simulink model "simulation"  (R2019a)
settings: Solver=ode45  StartTime=0.0  StopTime=300  FixedStep=Ts  RelTol=1e-3  EnableMultiTasking=on
values from neighbouring files (symbols this model uses):
  Ad = M22'    [VanLoan.m]    (also in initKalmanFilter.m = N(11:20, 11:20)')
  alfa1 = .2    (= 0.2)    [parameters.m]
  alfa2 = .2    (= 0.2)    [parameters.m]
  b1 = 0.1    [createModelFile.m]    (also in initCtrlPlantModel.m; parameters.m)
  b2 = 0.1    [createModelFile.m]    (also in initCtrlPlantModel.m; parameters.m)
  b3_nom = 0.1    [parameters.m]
  b4_nom = 0.1    [parameters.m]
  b5 = 0.1    [createModelFile.m]    (also in initCtrlPlantModel.m; parameters.m)
  Bd = N12    [VanLoan.m]
  C_D_Re_GNARC = C_C_Re    [start_up.m]
  Cc = [ ... (first row only)    [initCtrlPlantModel.m]    (also in initKFs.m = ctrlPlantModel.C; initTask1.m = ctrlPlantModel.C)
  D_D_Re_GNARC = D_C_Re    [start_up.m]
  k1 = 0.15    [createModelFile.m]    (also in initCtrlPlantModel.m; parameters.m)
  k3_nom = .1    (= 0.1)    [parameters.m]
  k4_nom = .1    (= 0.1)    [parameters.m]
  m1 = 1    [parameters.m]
  m2 = 1    [parameters.m]
  m3 = 1    [parameters.m]
  m4 = 1    [parameters.m]
  P0 = diag([1, 1, 1, 1, 10, 10, 10, 10, 1, 1].^2)    [initKFs.m]    (also in initTask1.m = diag([1e-3, 1e-3, 1e-3, 1e-3, 1e-3, 1e-3, 1e-3, 1e-3, 1e-3, ; initTask2.m = diag([1e-3, 1e-3, 1e-3, 1e-3, 1e-3, 1e-3, 1e-3, 1e-3, 1e-3, )
  probThreshold = 1e-6    (= 1e-06)    [initTask2.m]
  Qd = M22'*M12    [VanLoan.m]    (also in initKalmanFilter.m = Ad*N(1:10, 11:20))
  Rd = R / Ts    [initKFs.m]    (also in initTask1.m = Rn / Ts; initTask2.m = Rn / Ts)
  Ts = .001    (= 0.001)    [parameters.m]
  x0 = [0; 0; 0; 0; 0; 0; 0; 0; 0; 0;]    [initKFs.m]    (also in initTask1.m; initTask2.m)
undefined symbols (not defined in the file or in its folder): A_D_Re_GNARC, Ad1, Ad2, Ad3, B_D_Re_GNARC, Bd1, Bd2, Bd3, L1, L2, L3, P1, P2, P3, Qd1, Qd2, Qd3
libraries: simulink x4
settings Model: Creator=VAHiD  LastModifiedBy=marti
settings DataIOCC: LimitDataPoints=on  SaveFormat=Array  ReturnWorkspaceOutputs=off
settings OptimizationCC: ExpressionDepthLimit=2147483647  LifeSpan=inf
settings DebuggingCC: UnderspecifiedInitializationDetection=Classic  MergeDetectMultiDrivingBlocksExec=none  SolverPrmCheckMsg=warning  FcnCallInpInsideContextMsg=warning  StateNameClashWarn=warning  PregeneratedLibrarySubsystemCodeDiagnostic=none  SFUnexpectedBacktrackingDiag=warning  SFNoUnconditionalDefaultTransitionDiag=warning  SFExecutionAtInitializationDiag=none  ArithmeticOperatorsInVariantConditions=warning
settings HardwareCC: ProdBitPerPointer=32  ProdBitPerSizeT=32  ProdBitPerPtrDiffT=32  ProdLargestAtomicFloat=None  ProdIntDivRoundTo=Undefined  ProdEndianess=Unspecified  ProdWordSize=32  ProdHWDeviceType=32-bit Generic
settings ModelReferenceCC: PropagateSignalLabelsOutOfModel=off
settings SFSimCC: SimUseLocalCustomCode=off
settings RTWCC: RTWUseLocalCustomCode=off
settings CodeAppCC: StateflowObjectComments=on
settings GRTTargetCC: TargetLangStandard=C89/C90 (ANSI)  GeneratePreprocessorConditionals=Disable all  CombineOutputUpdateFcns=off  GRTInterface=on
settings ConfigComp: CovMetricSettings=dw  CovHtmlReporting=on  CovSaveCumulativeToWorkspaceVar=on  CovSaveSingleToWorkspaceVar=on  CovExternalEMLEnable=off

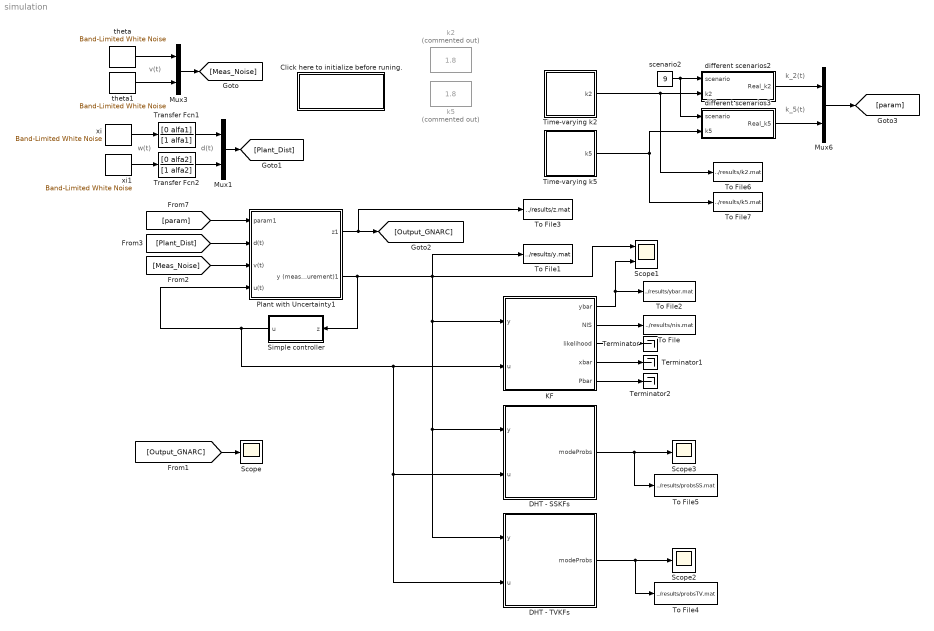
== system simulation ==
  note: w(t)
  note: v(t)
  note: d(t)
  note: k_2(t)
  note: k_5(t)
  Click here to initialize before runing. : Subsystem
      settings: OpenFcn=start_up
      mask Display: disp('Load\Parameters')
  DHT - SSKFs : Subsystem
  DHT - TVKFs : Subsystem
  KF : Subsystem
  Mux1 : Mux  Inputs=2
  Mux3 : Mux  Inputs=2
  Mux6 : Mux  Inputs=2
  Plant with Uncertainty1 : Subsystem
  Scope : Scope
  Scope1 : Scope  NumInputPorts=2
  Scope2 : Scope
  Scope3 : Scope
  Simple controller : Subsystem
  Terminator : Terminator
  Terminator1 : Terminator
  Terminator2 : Terminator
  Time-varying k2 : Subsystem
  Time-varying k5 : Subsystem
  To File : ToFile  Filename=../results/nis.mat  MatrixName=nis
  To File1 : ToFile  Filename=../results/y.mat  MatrixName=y
  To File2 : ToFile  Filename=../results/ybar.mat  MatrixName=ybar
  To File3 : ToFile  Filename=../results/z.mat  MatrixName=z
  To File4 : ToFile  Filename=../results/probsTV.mat  MatrixName=probsTV
  To File5 : ToFile  Filename=../results/probsSS.mat  MatrixName=probsSS
  To File6 : ToFile  Filename=../results/k2.mat  MatrixName=k2
  To File7 : ToFile  Filename=../results/k5.mat  MatrixName=k5
  Transfer Fcn1 : TransferFcn  Numerator=[0 alfa1]  Denominator=[1 alfa1]
  Transfer Fcn2 : TransferFcn  Numerator=[0 alfa2]  Denominator=[1 alfa2]
  different scenarios2 : Subsystem
  different scenarios3 : Subsystem
  k2 : Constant  Commented=on  Value=1.8
  k5 : Constant  Commented=on  Value=1.8
  scenario2 : Constant  Value=9
  theta : simulink/Sources/Band-Limited White Noise  Cov=TH1  Ts=Ts  seed=1
  theta1 : simulink/Sources/Band-Limited White Noise  Cov=TH2  Ts=Ts  seed=2
  xi : simulink/Sources/Band-Limited White Noise  Cov=XI1  Ts=Ts  seed=3
  xi1 : simulink/Sources/Band-Limited White Noise  Cov=XI2  Ts=Ts  seed=4
  wires:
  Mux3/1 -> [Meas_Noise]
  theta/1 -> Mux3/1
  theta1/1 -> Mux3/2
  Mux1/1 -> [Plant_Dist]
  xi/1 -> Transfer Fcn1/1
  xi1/1 -> Transfer Fcn2/1
  Transfer Fcn1/1 -> Mux1/1
  Transfer Fcn2/1 -> Mux1/2
  scenario2/1 -> different scenarios2/1(scenario), different scenarios3/1(scenario)
  different scenarios3/1(Real_k5) -> Mux6/2
  different scenarios2/1(Real_k2) -> Mux6/1
  Mux6/1 -> [param]
  [param] -> Plant with Uncertainty1/1(param1)
  [Plant_Dist] -> Plant with Uncertainty1/2(d(t))
  [Meas_Noise] -> Plant with Uncertainty1/3(v(t))
  Plant with Uncertainty1/1(z1) -> To File3/1, [Output_GNARC]
  Simple controller/1(u) -> DHT - SSKFs/2(u), DHT - TVKFs/2(u), KF/2(u), Plant with Uncertainty1/4(u(t))
  [Output_GNARC] -> Scope/1
  Plant with Uncertainty1/2(y (measurement)1) -> Simple controller/1(z), DHT - TVKFs/1(y), DHT - SSKFs/1(y), KF/1(y), Scope1/1, To File1/1
  KF/4(xbar) -> Terminator1/1
  KF/3(likelihood) -> Terminator/1
  KF/5(Pbar) -> Terminator2/1
  KF/1(ybar) -> To File2/1, Scope1/2
  KF/2(NIS) -> To File/1
  DHT - TVKFs/1(modeProbs) -> Scope2/1, To File4/1
  DHT - SSKFs/1(modeProbs) -> To File5/1, Scope3/1
  Time-varying k2/1(k2) -> To File6/1, different scenarios2/2(k2)
  Time-varying k5/1(k5) -> To File7/1, different scenarios3/2(k5)

== system simulation/Click here to initialize before runing. ==

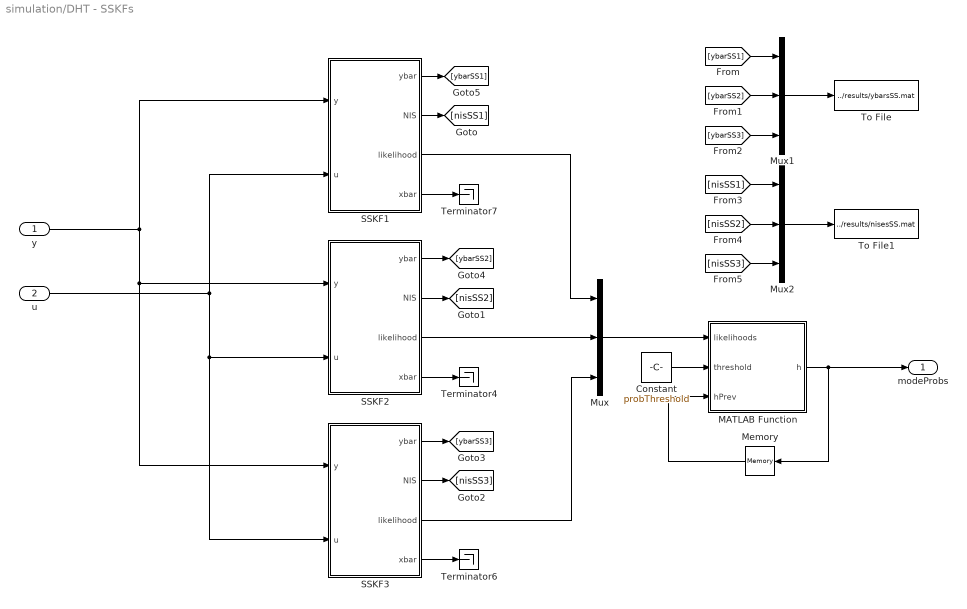
== system simulation/DHT - SSKFs ==
  y : Inport
  u : Inport  Port=2
  Constant : Constant  Value=probThreshold
  MATLAB Function : MATLAB Function  TreatAsAtomicUnit=on
  Memory : Memory  InitialCondition=[1/3, 1/3, 1/3]
  Mux : Mux  Inputs=3
  Mux1 : Mux  Inputs=3
  Mux2 : Mux  Inputs=3
  SSKF1 : Subsystem
  SSKF2 : Subsystem
  SSKF3 : Subsystem
  Terminator4 : Terminator
  Terminator6 : Terminator
  Terminator7 : Terminator
  To File : ToFile  Filename=../results/ybarsSS.mat  MatrixName=ybarsSS
  To File1 : ToFile  Filename=../results/nisesSS.mat  MatrixName=nisesSS
  modeProbs : Outport
  wires:
  u/1 -> SSKF3/2(u), SSKF2/2(u), SSKF1/2(u)
  y/1 -> SSKF3/1(y), SSKF2/1(y), SSKF1/1(y)
  SSKF1/3(likelihood) -> Mux/1
  SSKF2/3(likelihood) -> Mux/2
  SSKF3/3(likelihood) -> Mux/3
  SSKF2/1(ybar) -> [ybarSS2]
  SSKF1/1(ybar) -> [ybarSS1]
  SSKF1/2(NIS) -> [nisSS1]
  SSKF2/2(NIS) -> [nisSS2]
  SSKF3/1(ybar) -> [ybarSS3]
  SSKF2/4(xbar) -> Terminator4/1
  SSKF3/4(xbar) -> Terminator6/1
  SSKF1/4(xbar) -> Terminator7/1
  SSKF3/2(NIS) -> [nisSS3]
  Constant/1 -> MATLAB Function/2(threshold)
  MATLAB Function/1(h) -> modeProbs/1, Memory/1
  Memory/1 -> MATLAB Function/3(hPrev)
  Mux/1 -> MATLAB Function/1(likelihoods)
  [ybarSS1] -> Mux1/1
  [ybarSS2] -> Mux1/2
  [ybarSS3] -> Mux1/3
  Mux1/1 -> To File/1
  [nisSS2] -> Mux2/2
  [nisSS3] -> Mux2/3
  [nisSS1] -> Mux2/1
  Mux2/1 -> To File1/1

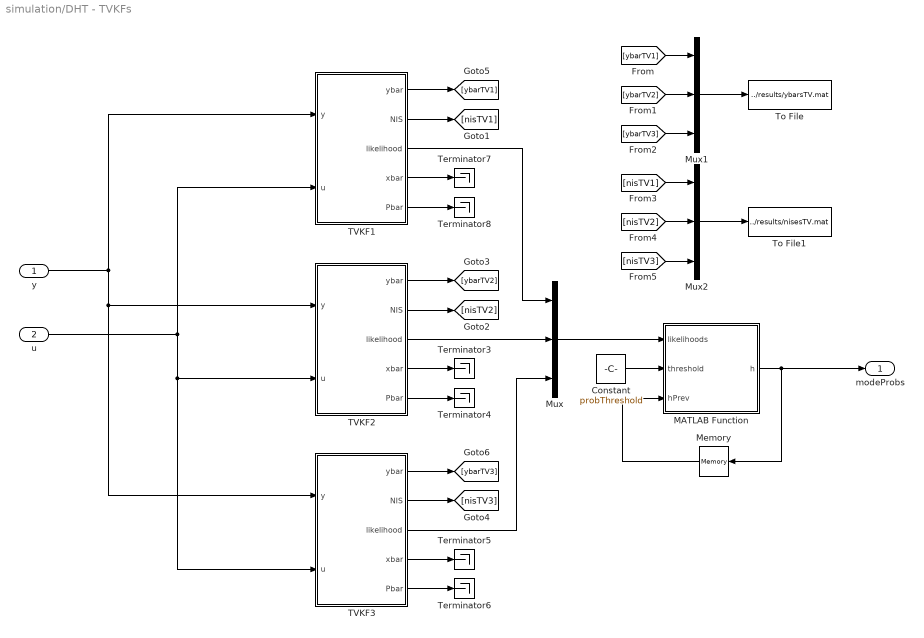
== system simulation/DHT - TVKFs ==
  y : Inport
  u : Inport  Port=2
  Constant : Constant  Value=probThreshold
  MATLAB Function : MATLAB Function  TreatAsAtomicUnit=on
  Memory : Memory  InitialCondition=[1/3, 1/3, 1/3]
  Mux : Mux  Inputs=3
  Mux1 : Mux  Inputs=3
  Mux2 : Mux  Inputs=3
  TVKF1 : Subsystem
  TVKF2 : Subsystem
  TVKF3 : Subsystem
  Terminator{3..8} (6 alike) : Terminator
  To File : ToFile  Filename=../results/ybarsTV.mat  MatrixName=ybarsTV
  To File1 : ToFile  Filename=../results/nisesTV.mat  MatrixName=nisesTV
  modeProbs : Outport
  wires:
  u/1 -> TVKF3/2(u), TVKF2/2(u), TVKF1/2(u)
  y/1 -> TVKF3/1(y), TVKF2/1(y), TVKF1/1(y)
  TVKF1/3(likelihood) -> Mux/1
  TVKF2/3(likelihood) -> Mux/2
  TVKF3/3(likelihood) -> Mux/3
  Mux/1 -> MATLAB Function/1(likelihoods)
  MATLAB Function/1(h) -> modeProbs/1, Memory/1
  Memory/1 -> MATLAB Function/3(hPrev)
  TVKF3/1(ybar) -> [ybarTV3]
  TVKF2/1(ybar) -> [ybarTV2]
  TVKF1/1(ybar) -> [ybarTV1]
  TVKF1/2(NIS) -> [nisTV1]
  TVKF2/2(NIS) -> [nisTV2]
  TVKF3/2(NIS) -> [nisTV3]
  TVKF2/4(xbar) -> Terminator3/1
  TVKF2/5(Pbar) -> Terminator4/1
  TVKF3/4(xbar) -> Terminator5/1
  TVKF3/5(Pbar) -> Terminator6/1
  TVKF1/4(xbar) -> Terminator7/1
  TVKF1/5(Pbar) -> Terminator8/1
  Constant/1 -> MATLAB Function/2(threshold)
  Mux1/1 -> To File/1
  [nisTV1] -> Mux2/1
  [ybarTV3] -> Mux1/3
  [ybarTV1] -> Mux1/1
  [nisTV3] -> Mux2/3
  Mux2/1 -> To File1/1
  [ybarTV2] -> Mux1/2
  [nisTV2] -> Mux2/2

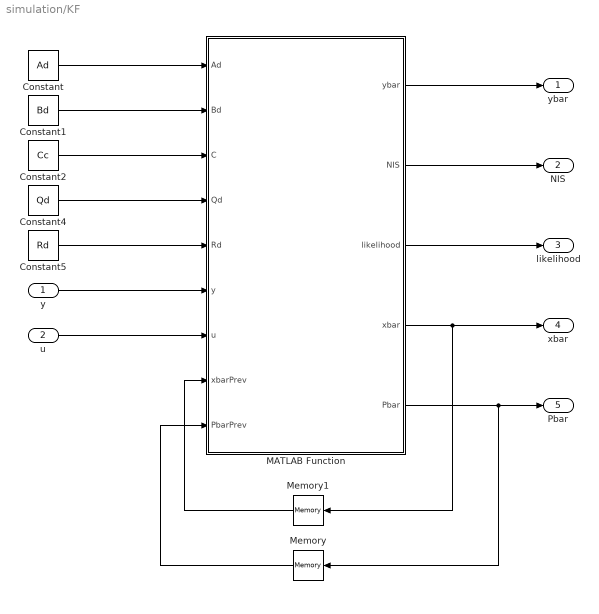
== system simulation/KF ==
  y : Inport
  u : Inport  Port=2
  Constant : Constant  Value=Ad
  Constant1 : Constant  Value=Bd
  Constant2 : Constant  Value=Cc
  Constant4 : Constant  Value=Qd
  Constant5 : Constant  Value=Rd
  MATLAB Function : MATLAB Function  TreatAsAtomicUnit=on
  Memory : Memory  InitialCondition=P0
  Memory1 : Memory  InitialCondition=x0
  ybar : Outport
  NIS : Outport  Port=2
  likelihood : Outport  Port=3
  xbar : Outport  Port=4
  Pbar : Outport  Port=5
  wires:
  y/1 -> MATLAB Function/6(y)
  u/1 -> MATLAB Function/7(u)
  MATLAB Function/1(ybar) -> ybar/1
  Constant2/1 -> MATLAB Function/3(C)
  Constant1/1 -> MATLAB Function/2(Bd)
  Constant/1 -> MATLAB Function/1(Ad)
  Constant4/1 -> MATLAB Function/4(Qd)
  Constant5/1 -> MATLAB Function/5(Rd)
  MATLAB Function/2(NIS) -> NIS/1
  MATLAB Function/3(likelihood) -> likelihood/1
  MATLAB Function/4(xbar) -> Memory1/1, xbar/1
  MATLAB Function/5(Pbar) -> Memory/1, Pbar/1
  Memory1/1 -> MATLAB Function/8(xbarPrev)
  Memory/1 -> MATLAB Function/9(PbarPrev)

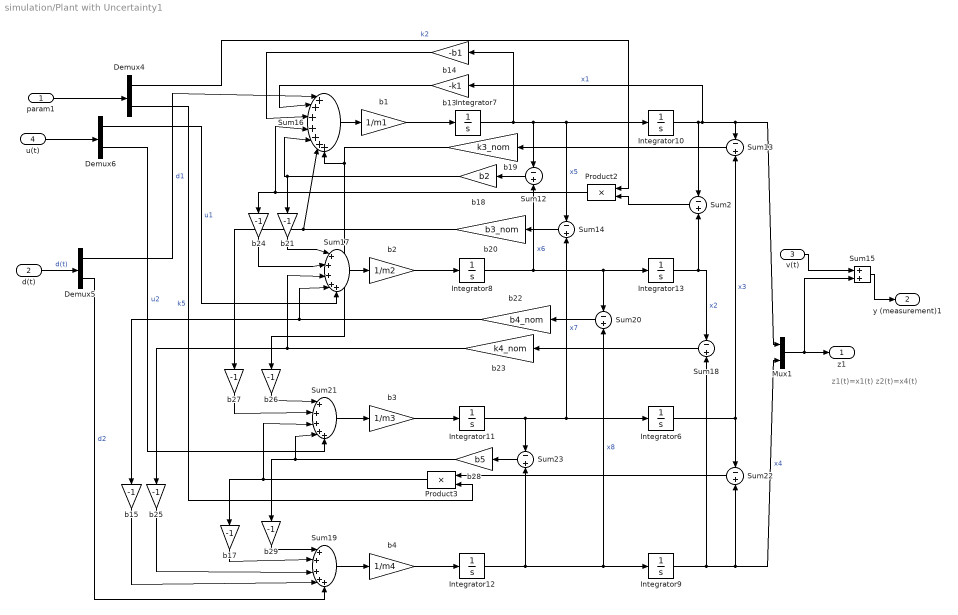
== system simulation/Plant with Uncertainty1 ==
  note: z1(t)=x1(t)
      | z2(t)=x4(t)
  param1 : Inport
  d(t) : Inport  Port=2
  v(t) : Inport  Port=3
  u(t) : Inport  Port=4
  Demux4 : Demux  Outputs=2
  Demux5 : Demux  Outputs=2
  Demux6 : Demux  Outputs=2
  Integrator{6..13} (8 alike) : Integrator
  Mux1 : Mux  Inputs=2
  Product2 : Product  SaturateOnIntegerOverflow=on  InputSameDT=on  OutDataTypeStr=Inherit: Same as first input
  Product3 : Product  SaturateOnIntegerOverflow=on  InputSameDT=on  OutDataTypeStr=Inherit: Same as first input
  Sum{2,12..14,18,20,22..23} (8 alike) : Sum  Inputs=-+  SaturateOnIntegerOverflow=on  InputSameDT=on  OutDataTypeStr=Inherit: Same as first input
  Sum15 : Sum  SaturateOnIntegerOverflow=on  InputSameDT=on  OutDataTypeStr=Inherit: Same as first input
  Sum16 : Sum  Inputs=|+++++++  SaturateOnIntegerOverflow=on  InputSameDT=on  OutDataTypeStr=Inherit: Same as first input
  Sum17 : Sum  Inputs=|+++++  SaturateOnIntegerOverflow=on  InputSameDT=on  OutDataTypeStr=Inherit: Same as first input
  Sum19 : Sum  Inputs=|+++++  SaturateOnIntegerOverflow=on  InputSameDT=on  OutDataTypeStr=Inherit: Same as first input
  Sum21 : Sum  Inputs=|+++++  SaturateOnIntegerOverflow=on  InputSameDT=on  OutDataTypeStr=Inherit: Same as first input
  b1 : Gain  Gain=1/m1  SaturateOnIntegerOverflow=on  OutDataTypeStr=Inherit: Same as input  ParamDataTypeStr=Inherit: Same as input
  b13 : Gain  Gain=-k1  SaturateOnIntegerOverflow=on  OutDataTypeStr=Inherit: Same as input  ParamDataTypeStr=Inherit: Same as input
  b14 : Gain  Gain=-b1  SaturateOnIntegerOverflow=on  OutDataTypeStr=Inherit: Same as input  ParamDataTypeStr=Inherit: Same as input
  b{15,17,21,24..27,29} (8 alike) : Gain  Gain=-1  SaturateOnIntegerOverflow=on  OutDataTypeStr=Inherit: Same as input  ParamDataTypeStr=Inherit: Same as input
  b18 : Gain  Gain=b2  SaturateOnIntegerOverflow=on  OutDataTypeStr=Inherit: Same as input  ParamDataTypeStr=Inherit: Same as input
  b19 : Gain  Gain=k3_nom  SaturateOnIntegerOverflow=on  OutDataTypeStr=Inherit: Same as input  ParamDataTypeStr=Inherit: Same as input
  b2 : Gain  Gain=1/m2  SaturateOnIntegerOverflow=on  OutDataTypeStr=Inherit: Same as input  ParamDataTypeStr=Inherit: Same as input
  b20 : Gain  Gain=b3_nom  SaturateOnIntegerOverflow=on  OutDataTypeStr=Inherit: Same as input  ParamDataTypeStr=Inherit: Same as input
  b22 : Gain  Gain=b4_nom  SaturateOnIntegerOverflow=on  OutDataTypeStr=Inherit: Same as input  ParamDataTypeStr=Inherit: Same as input
  b23 : Gain  Gain=k4_nom  SaturateOnIntegerOverflow=on  OutDataTypeStr=Inherit: Same as input  ParamDataTypeStr=Inherit: Same as input
  b28 : Gain  Gain=b5  SaturateOnIntegerOverflow=on  OutDataTypeStr=Inherit: Same as input  ParamDataTypeStr=Inherit: Same as input
  b3 : Gain  Gain=1/m3  SaturateOnIntegerOverflow=on  OutDataTypeStr=Inherit: Same as input  ParamDataTypeStr=Inherit: Same as input
  b4 : Gain  Gain=1/m4  SaturateOnIntegerOverflow=on  OutDataTypeStr=Inherit: Same as input  ParamDataTypeStr=Inherit: Same as input
  z1 : Outport
  y (measurement)1 : Outport  Port=2
  wires:
  Sum15/1 -> y (measurement)1/1
  v(t)/1 -> Sum15/1
  param1/1 -> Demux4/1
  Mux1/1 -> Sum15/2, z1/1
  d(t)/1 -> Demux5/1  "d(t)"
  u(t)/1 -> Demux6/1
  b25/1 -> Sum19/3
  b15/1 -> Sum19/4
  Demux5/2 -> Sum19/5  "d2"
  Integrator7/1 -> b14/1, Sum12/1, Integrator10/1, Sum14/1  "x5"
  Integrator10/1 -> b13/1, Sum13/1, Mux1/1, Sum2/1  "x1"
  Integrator8/1 -> Sum12/2, Integrator13/1, Sum20/1  "x6"
  Integrator11/1 -> Integrator6/1, Sum14/2, Sum23/1  "x7"
  Integrator12/1 -> Integrator9/1, Sum20/2, Sum23/2  "x8"
  Demux5/1 -> Sum16/1  "d1"
  b13/1 -> Sum16/2
  b14/1 -> Sum16/3
  Integrator13/1 -> Sum2/2, Sum18/1  "x2"
  Sum2/1 -> Product2/2
  Demux4/1 -> Product2/1  "k2"
  Sum12/1 -> b18/1
  b18/1 -> Sum16/5, b21/1
  Integrator6/1 -> Sum13/2, Sum22/1  "x3"
  Sum13/1 -> b19/1
  Sum14/1 -> b20/1
  b20/1 -> Sum16/6, b27/1
  Sum16/1 -> b1/1
  Product2/1 -> Sum16/4, b24/1
  Integrator9/1 -> Sum18/2, Sum22/2, Mux1/2  "x4"
  Sum18/1 -> b23/1
  b23/1 -> Sum17/3, b25/1
  Sum17/1 -> b2/1
  Sum20/1 -> b22/1
  b22/1 -> Sum17/4, b15/1
  b21/1 -> Sum17/1
  b24/1 -> Sum17/2
  Demux6/1 -> Sum17/5  "u1"
  Sum21/1 -> b3/1
  b19/1 -> Sum16/7, b26/1
  b26/1 -> Sum21/1
  b27/1 -> Sum21/2
  Sum22/1 -> Product3/1
  Product3/1 -> Sum21/3, b17/1
  Demux4/2 -> Product3/2  "k5"
  Sum23/1 -> b28/1
  b28/1 -> Sum21/4, b29/1
  Demux6/2 -> Sum21/5  "u2"
  Sum19/1 -> b4/1
  b17/1 -> Sum19/2
  b29/1 -> Sum19/1
  b1/1 -> Integrator7/1
  b2/1 -> Integrator8/1
  b3/1 -> Integrator11/1
  b4/1 -> Integrator12/1

== system simulation/Simple controller ==
  z : Inport
  Discrete mu-controller 1 : DiscreteStateSpace  Description=disp('sss')  A=A_D_Re_GNARC  B=B_D_Re_GNARC  C=C_D_Re_GNARC  D=D_D_Re_GNARC  SampleTime=Ts
  u : Outport
  wires:
  z/1 -> Discrete mu-controller 1/1
  Discrete mu-controller 1/1 -> u/1

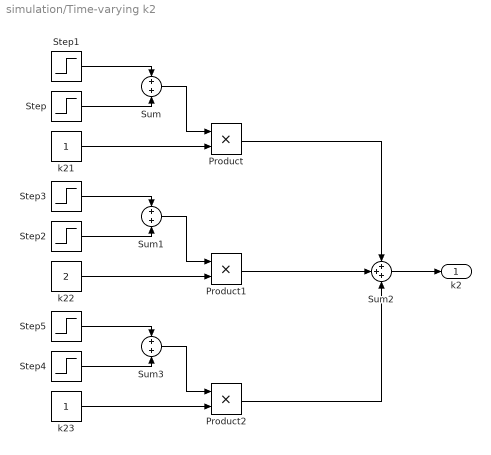
== system simulation/Time-varying k2 ==
  Product : Product
  Product1 : Product
  Product2 : Product
  Step : Step  Time=100  After=-1  SampleTime=0
  Step1 : Step  SampleTime=0
  Step2 : Step  Time=300  After=-1  SampleTime=0
  Step3 : Step  Time=100  SampleTime=0
  Step4 : Step  Time=300  After=-1  SampleTime=0
  Step5 : Step  Time=300  SampleTime=0
  Sum : Sum  Inputs=+|+
  Sum1 : Sum  Inputs=+|+
  Sum2 : Sum  Inputs=+++
  Sum3 : Sum  Inputs=+|+
  k21 : Constant
  k22 : Constant  Value=2
  k23 : Constant
  k2 : Outport
  wires:
  k21/1 -> Product/2
  Sum/1 -> Product/1
  Step1/1 -> Sum/1
  Step/1 -> Sum/2
  Step3/1 -> Sum1/1
  Sum1/1 -> Product1/1
  Step2/1 -> Sum1/2
  k22/1 -> Product1/2
  Sum3/1 -> Product2/1
  Step4/1 -> Sum3/2
  k23/1 -> Product2/2
  Step5/1 -> Sum3/1
  Product1/1 -> Sum2/2
  Product2/1 -> Sum2/3
  Product/1 -> Sum2/1
  Sum2/1 -> k2/1

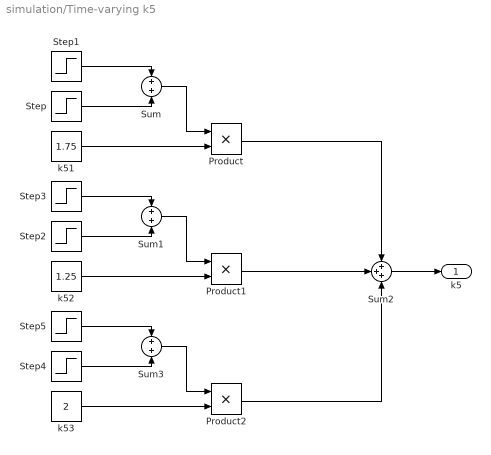
== system simulation/Time-varying k5 ==
  Product : Product
  Product1 : Product
  Product2 : Product
  Step : Step  Time=100  After=-1  SampleTime=0
  Step1 : Step  SampleTime=0
  Step2 : Step  Time=200  After=-1  SampleTime=0
  Step3 : Step  Time=100  SampleTime=0
  Step4 : Step  Time=300  After=-1  SampleTime=0
  Step5 : Step  Time=200  SampleTime=0
  Sum : Sum  Inputs=+|+
  Sum1 : Sum  Inputs=+|+
  Sum2 : Sum  Inputs=+++
  Sum3 : Sum  Inputs=+|+
  k51 : Constant  Value=1.75
  k52 : Constant  Value=1.25
  k53 : Constant  Value=2
  k5 : Outport
  wires:
  k51/1 -> Product/2
  Sum/1 -> Product/1
  Step1/1 -> Sum/1
  Step/1 -> Sum/2
  Step3/1 -> Sum1/1
  Sum1/1 -> Product1/1
  Step2/1 -> Sum1/2
  k52/1 -> Product1/2
  Sum3/1 -> Product2/1
  Step4/1 -> Sum3/2
  k53/1 -> Product2/2
  Step5/1 -> Sum3/1
  Product1/1 -> Sum2/2
  Product2/1 -> Sum2/3
  Product/1 -> Sum2/1
  Sum2/1 -> k5/1

== system simulation/different scenarios2 ==
  scenario : Inport
  k2 : Inport  Port=2
  GNARC : Sin  Amplitude=.75  Bias=1  Frequency=2*pi/700  Phase=-pi/2  SampleTime=0
  LNARC1 : Sin  Amplitude=.875  Bias=1.625  Frequency=2*pi/700  Phase=-pi/2  SampleTime=0
  LNARC2 : Sin  Amplitude=.55/2  Bias=.775  Frequency=2*pi/700  Phase=-pi/2  SampleTime=0
  LNARC3 : Sin  Amplitude=.75/2  Bias=1.4250  Frequency=2*pi/700  Phase=-pi/2  SampleTime=0
  LNARC4 : Sin  Amplitude=.15/2  Bias=.325  Frequency=2*pi/700  Phase=-pi/2  SampleTime=0
  LNARC5 : Sin  Amplitude=.15  Bias=.55  Frequency=2*pi/700  Phase=-pi/2  SampleTime=0
  LNARC6 : Sin  Amplitude=.45/2  Bias=.925  Frequency=2*pi/700  Phase=-pi/2  SampleTime=0
  LNARC7 : Sin  Amplitude=.30  Bias=1.45  Frequency=2*pi/700  Phase=-pi/2  SampleTime=0
  Multiport Switch : MultiPortSwitch  Inputs=9
  Real_k2 : Outport
  wires:
  Multiport Switch/1 -> Real_k2/1
  scenario/1 -> Multiport Switch/1
  LNARC3/1 -> Multiport Switch/4
  LNARC6/1 -> Multiport Switch/7
  LNARC7/1 -> Multiport Switch/8
  LNARC5/1 -> Multiport Switch/6
  LNARC4/1 -> Multiport Switch/5
  LNARC1/1 -> Multiport Switch/2
  LNARC2/1 -> Multiport Switch/3
  k2/1 -> Multiport Switch/10
  GNARC/1 -> Multiport Switch/9

== system simulation/different scenarios3 ==
  scenario : Inport
  k5 : Inport  Port=2
  GNARC : Sin  Amplitude=1.6  Bias=1.8  Frequency=2*pi/700  Phase=-pi/2  SampleTime=0
  LNARC1 : Sin  Amplitude=.8  Bias=1.7  Frequency=2*pi/700  Phase=-3*pi/2  SampleTime=0
  LNARC2 : Sin  Amplitude=.8  Bias=2.6  Frequency=2*pi/700  Phase=-pi/2  SampleTime=0
  LNARC3 : Sin  Amplitude=.8  Bias=2.6  Frequency=2*pi/700  Phase=-pi/2  SampleTime=0
  LNARC{4..7} (4 alike) : Sin  Amplitude=.8  Bias=1  Frequency=2*pi/700  Phase=-pi/2  SampleTime=0
  Multiport Switch : MultiPortSwitch  Inputs=9
  Real_k5 : Outport
  wires:
  LNARC5/1 -> Multiport Switch/6
  LNARC7/1 -> Multiport Switch/8
  LNARC6/1 -> Multiport Switch/7
  LNARC3/1 -> Multiport Switch/4
  scenario/1 -> Multiport Switch/1
  Multiport Switch/1 -> Real_k5/1
  k5/1 -> Multiport Switch/10
  GNARC/1 -> Multiport Switch/9
  LNARC1/1 -> Multiport Switch/2
  LNARC2/1 -> Multiport Switch/3
  LNARC4/1 -> Multiport Switch/5

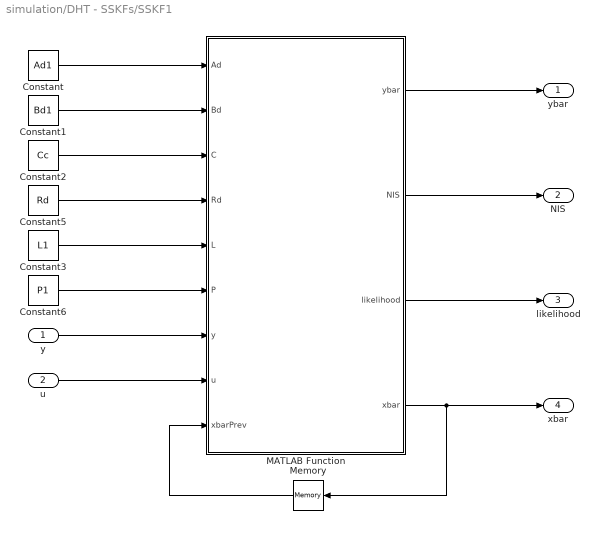
== system simulation/DHT - SSKFs/SSKF1 ==
  y : Inport
  u : Inport  Port=2
  Constant : Constant  Value=Ad1
  Constant1 : Constant  Value=Bd1
  Constant2 : Constant  Value=Cc
  Constant3 : Constant  Value=L1
  Constant5 : Constant  Value=Rd
  Constant6 : Constant  Value=P1
  MATLAB Function : MATLAB Function  TreatAsAtomicUnit=on
  Memory : Memory  InitialCondition=x0
  ybar : Outport
  NIS : Outport  Port=2
  likelihood : Outport  Port=3
  xbar : Outport  Port=4
  wires:
  y/1 -> MATLAB Function/7(y)
  u/1 -> MATLAB Function/8(u)
  MATLAB Function/1(ybar) -> ybar/1
  Constant2/1 -> MATLAB Function/3(C)
  Constant1/1 -> MATLAB Function/2(Bd)
  Constant/1 -> MATLAB Function/1(Ad)
  Constant5/1 -> MATLAB Function/4(Rd)
  MATLAB Function/2(NIS) -> NIS/1
  MATLAB Function/3(likelihood) -> likelihood/1
  MATLAB Function/4(xbar) -> xbar/1, Memory/1
  Constant3/1 -> MATLAB Function/5(L)
  Constant6/1 -> MATLAB Function/6(P)
  Memory/1 -> MATLAB Function/9(xbarPrev)

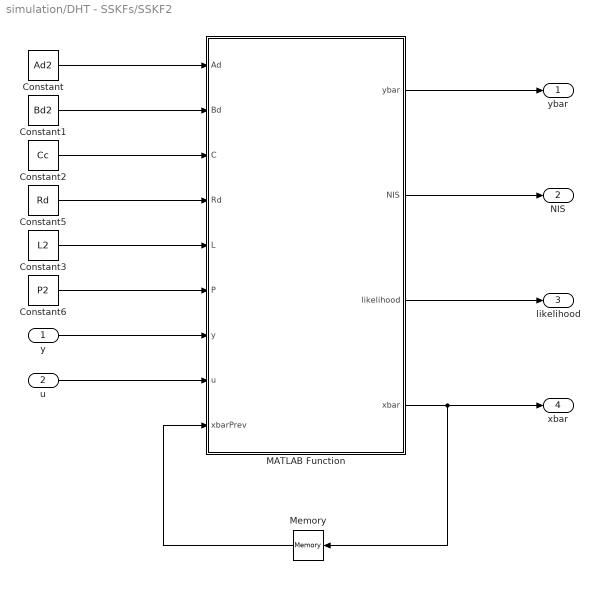
== system simulation/DHT - SSKFs/SSKF2 ==
  y : Inport
  u : Inport  Port=2
  Constant : Constant  Value=Ad2
  Constant1 : Constant  Value=Bd2
  Constant2 : Constant  Value=Cc
  Constant3 : Constant  Value=L2
  Constant5 : Constant  Value=Rd
  Constant6 : Constant  Value=P2
  MATLAB Function : MATLAB Function  TreatAsAtomicUnit=on
  Memory : Memory  InitialCondition=x0
  ybar : Outport
  NIS : Outport  Port=2
  likelihood : Outport  Port=3
  xbar : Outport  Port=4
  wires:
  y/1 -> MATLAB Function/7(y)
  u/1 -> MATLAB Function/8(u)
  MATLAB Function/1(ybar) -> ybar/1
  Constant2/1 -> MATLAB Function/3(C)
  Constant1/1 -> MATLAB Function/2(Bd)
  Constant/1 -> MATLAB Function/1(Ad)
  Constant5/1 -> MATLAB Function/4(Rd)
  MATLAB Function/2(NIS) -> NIS/1
  MATLAB Function/3(likelihood) -> likelihood/1
  MATLAB Function/4(xbar) -> xbar/1, Memory/1
  Constant3/1 -> MATLAB Function/5(L)
  Constant6/1 -> MATLAB Function/6(P)
  Memory/1 -> MATLAB Function/9(xbarPrev)

== system simulation/DHT - SSKFs/SSKF3 ==
  y : Inport
  u : Inport  Port=2
  Constant : Constant  Value=Ad3
  Constant1 : Constant  Value=Bd3
  Constant2 : Constant  Value=Cc
  Constant3 : Constant  Value=L3
  Constant5 : Constant  Value=Rd
  Constant6 : Constant  Value=P3
  MATLAB Function : MATLAB Function  TreatAsAtomicUnit=on
  Memory : Memory  InitialCondition=x0
  ybar : Outport
  NIS : Outport  Port=2
  likelihood : Outport  Port=3
  xbar : Outport  Port=4
  wires:
  y/1 -> MATLAB Function/7(y)
  u/1 -> MATLAB Function/8(u)
  MATLAB Function/1(ybar) -> ybar/1
  Constant2/1 -> MATLAB Function/3(C)
  Constant1/1 -> MATLAB Function/2(Bd)
  Constant/1 -> MATLAB Function/1(Ad)
  Constant5/1 -> MATLAB Function/4(Rd)
  MATLAB Function/2(NIS) -> NIS/1
  MATLAB Function/3(likelihood) -> likelihood/1
  MATLAB Function/4(xbar) -> xbar/1, Memory/1
  Constant3/1 -> MATLAB Function/5(L)
  Constant6/1 -> MATLAB Function/6(P)
  Memory/1 -> MATLAB Function/9(xbarPrev)

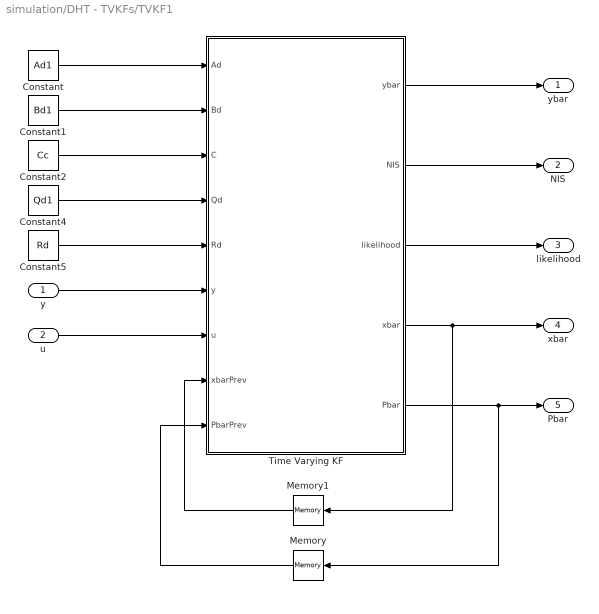
== system simulation/DHT - TVKFs/TVKF1 ==
  y : Inport
  u : Inport  Port=2
  Constant : Constant  Value=Ad1
  Constant1 : Constant  Value=Bd1
  Constant2 : Constant  Value=Cc
  Constant4 : Constant  Value=Qd1
  Constant5 : Constant  Value=Rd
  Memory : Memory  InitialCondition=P0
  Memory1 : Memory  InitialCondition=x0
  Time Varying KF : MATLAB Function  TreatAsAtomicUnit=on
  ybar : Outport
  NIS : Outport  Port=2
  likelihood : Outport  Port=3
  xbar : Outport  Port=4
  Pbar : Outport  Port=5
  wires:
  y/1 -> Time Varying KF/6(y)
  u/1 -> Time Varying KF/7(u)
  Time Varying KF/1(ybar) -> ybar/1
  Constant2/1 -> Time Varying KF/3(C)
  Constant1/1 -> Time Varying KF/2(Bd)
  Constant/1 -> Time Varying KF/1(Ad)
  Constant4/1 -> Time Varying KF/4(Qd)
  Constant5/1 -> Time Varying KF/5(Rd)
  Time Varying KF/2(NIS) -> NIS/1
  Time Varying KF/3(likelihood) -> likelihood/1
  Time Varying KF/4(xbar) -> Memory1/1, xbar/1
  Time Varying KF/5(Pbar) -> Memory/1, Pbar/1
  Memory1/1 -> Time Varying KF/8(xbarPrev)
  Memory/1 -> Time Varying KF/9(PbarPrev)

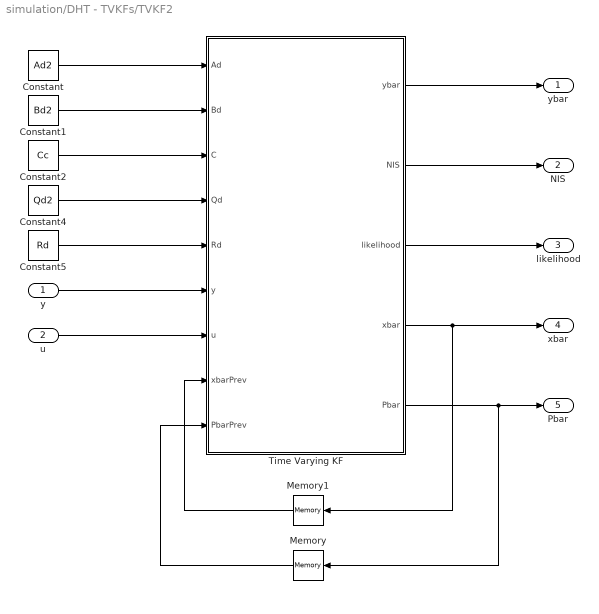
== system simulation/DHT - TVKFs/TVKF2 ==
  y : Inport
  u : Inport  Port=2
  Constant : Constant  Value=Ad2
  Constant1 : Constant  Value=Bd2
  Constant2 : Constant  Value=Cc
  Constant4 : Constant  Value=Qd2
  Constant5 : Constant  Value=Rd
  Memory : Memory  InitialCondition=P0
  Memory1 : Memory  InitialCondition=x0
  Time Varying KF : MATLAB Function  TreatAsAtomicUnit=on
  ybar : Outport
  NIS : Outport  Port=2
  likelihood : Outport  Port=3
  xbar : Outport  Port=4
  Pbar : Outport  Port=5
  wires:
  y/1 -> Time Varying KF/6(y)
  u/1 -> Time Varying KF/7(u)
  Time Varying KF/1(ybar) -> ybar/1
  Constant2/1 -> Time Varying KF/3(C)
  Constant1/1 -> Time Varying KF/2(Bd)
  Constant/1 -> Time Varying KF/1(Ad)
  Constant4/1 -> Time Varying KF/4(Qd)
  Constant5/1 -> Time Varying KF/5(Rd)
  Time Varying KF/2(NIS) -> NIS/1
  Time Varying KF/3(likelihood) -> likelihood/1
  Time Varying KF/4(xbar) -> Memory1/1, xbar/1
  Time Varying KF/5(Pbar) -> Memory/1, Pbar/1
  Memory1/1 -> Time Varying KF/8(xbarPrev)
  Memory/1 -> Time Varying KF/9(PbarPrev)

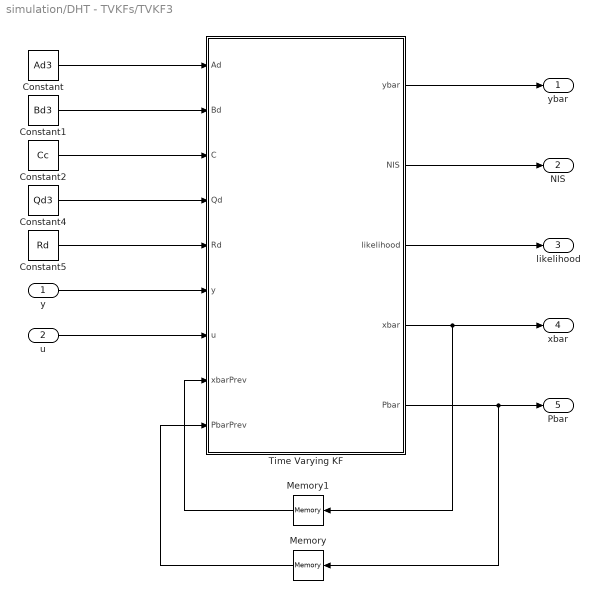
== system simulation/DHT - TVKFs/TVKF3 ==
  y : Inport
  u : Inport  Port=2
  Constant : Constant  Value=Ad3
  Constant1 : Constant  Value=Bd3
  Constant2 : Constant  Value=Cc
  Constant4 : Constant  Value=Qd3
  Constant5 : Constant  Value=Rd
  Memory : Memory  InitialCondition=P0
  Memory1 : Memory  InitialCondition=x0
  Time Varying KF : MATLAB Function  TreatAsAtomicUnit=on
  ybar : Outport
  NIS : Outport  Port=2
  likelihood : Outport  Port=3
  xbar : Outport  Port=4
  Pbar : Outport  Port=5
  wires:
  y/1 -> Time Varying KF/6(y)
  u/1 -> Time Varying KF/7(u)
  Time Varying KF/1(ybar) -> ybar/1
  Constant2/1 -> Time Varying KF/3(C)
  Constant1/1 -> Time Varying KF/2(Bd)
  Constant/1 -> Time Varying KF/1(Ad)
  Constant4/1 -> Time Varying KF/4(Qd)
  Constant5/1 -> Time Varying KF/5(Rd)
  Time Varying KF/2(NIS) -> NIS/1
  Time Varying KF/3(likelihood) -> likelihood/1
  Time Varying KF/4(xbar) -> Memory1/1, xbar/1
  Time Varying KF/5(Pbar) -> Memory/1, Pbar/1
  Memory1/1 -> Time Varying KF/8(xbarPrev)
  Memory/1 -> Time Varying KF/9(PbarPrev)

== matlab function simulation/KF/MATLAB Function ==
  data: Ad input; Bd input; C input; Qd input; Rd input; y input; u input; ybar output; NIS output; likelihood output; xbarPrev input; xbar output; PbarPrev input; Pbar output
function [ybar, NIS, likelihood, xbar, Pbar] = fcn(Ad, Bd, C, Qd, Rd, y, u, xbarPrev, PbarPrev)
n = size(xbarPrev, 1); 

I = eye(n);

xhat = Ad*xbarPrev + Bd*u; % Predicted states
Phat = Ad*PbarPrev*Ad' + Qd; % Predicted covariances
yhat = C*xhat; % Predicted measurements
v = y - yhat; % Innovation
S = C*Phat*C' + Rd; % Innovation covariance
W = Phat*C'*inv(S); % Kalman gain
xbar = xhat + W*v; % Update states
Pbar = (I - W*C)*Phat*(I - W*C)' + W*Rd*W'; % Update covariances
ybar = C*xbar; % Updated measurements
NIS = v'*inv(S)*v; % Normalized innovations squared

likelihood = exp(-1/2*NIS)/(sqrt((2*pi)^2*det(S)));
end

== matlab function simulation/DHT - SSKFs/SSKF1/MATLAB Function ==
  data: Ad input; Bd input; C input; Rd input; L input; P input; y input; u input; ybar output; NIS output; likelihood output; xbar output; xbarPrev input
function [ybar, NIS, likelihood, xbar] = fcn(Ad, Bd, C, Rd, ...
    L, P, y, u, xbarPrev) 

xhat = Ad*xbarPrev + Bd*u; % Predicted states
yhat = C*xhat; % Predicted measurements
v = y - yhat; % Innovation
S = C*P*C' + Rd; % Innovation covariance
xbar = xhat + L*v; % Update states
ybar = C*xbar; % Updated measurements
NIS = v'*inv(S)*v; % Normalized innovations squared

likelihood = exp(-1/2*NIS)/(sqrt((2*pi)^2*det(S)));
end

== matlab function simulation/DHT - SSKFs/SSKF2/MATLAB Function ==
  data: Ad input; Bd input; C input; Rd input; L input; P input; y input; u input; ybar output; NIS output; likelihood output; xbar output; xbarPrev input
function [ybar, NIS, likelihood, xbar] = fcn(Ad, Bd, C, Rd, ...
    L, P, y, u, xbarPrev)

xhat = Ad*xbarPrev + Bd*u; % Predicted states
yhat = C*xhat; % Predicted measurements
v = y - yhat; % Innovation
S = C*P*C' + Rd; % Innovation covariance
xbar = xhat + L*v; % Update states
ybar = C*xbar; % Updated measurements
NIS = v'*inv(S)*v; % Normalized innovations squared

likelihood = exp(-1/2*NIS)/(sqrt((2*pi)^2*det(S)));
end

== matlab function simulation/DHT - SSKFs/SSKF3/MATLAB Function ==
  data: Ad input; Bd input; C input; Rd input; L input; P input; y input; u input; ybar output; NIS output; likelihood output; xbar output; xbarPrev input
function [ybar, NIS, likelihood, xbar] = fcn(Ad, Bd, C, Rd, ...
    L, P, y, u, xbarPrev)
n = size(Ad, 1); 

xhat = Ad*xbarPrev + Bd*u; % Predicted states
yhat = C*xhat; % Predicted measurements
v = y - yhat; % Innovation
S = C*P*C' + Rd; % Innovation covariance
xbar = xhat + L*v; % Update states
ybar = C*xbar; % Updated measurements
NIS = v'*inv(S)*v; % Normalized innovations squared

likelihood = exp(-1/2*NIS)/(sqrt((2*pi)^2*det(S)));
end

== matlab function simulation/DHT - SSKFs/MATLAB Function ==
  data: likelihoods input; threshold input; hPrev input; h output
function h = likelihood(likelihoods, threshold, hPrev)
h = likelihoods.*hPrev;
h(h<threshold) = threshold;
h = h / sum(h);
end

== matlab function simulation/DHT - TVKFs/MATLAB Function ==
  data: likelihoods input; threshold input; hPrev input; h output
function h = likelihood(likelihoods, threshold, hPrev)
h = likelihoods.*hPrev;
h(h<threshold) = threshold;
h = h / sum(h);
end

== matlab function simulation/DHT - TVKFs/TVKF1/Time Varying KF ==
  data: Ad input; Bd input; C input; Qd input; Rd input; y input; u input; ybar output; NIS output; likelihood output; xbarPrev input; xbar output; PbarPrev input; Pbar output
function [ybar, NIS, likelihood, xbar, Pbar] = fcn(Ad, Bd, C, Qd, Rd, ...
    y, u, xbarPrev, PbarPrev)

n = size(xbarPrev, 1);
I = eye(n);

xhat = Ad*xbarPrev + Bd*u; % Predicted states
Phat = Ad*PbarPrev*Ad' + Qd; % Predicted covariances
yhat = C*xhat; % Predicted measurements
v = y - yhat; % Innovation
S = C*Phat*C' + Rd; % Innovation covariance
L = Phat*C'*inv(S); % Kalman gain
xbar = xhat + L*v; % Update states
Pbar = (I - L*C)*Phat*(I - L*C)' + L*Rd*L'; % Update covariances
ybar = C*xbar; % Updated measurements
NIS = v'*inv(S)*v; % Normalized innovations squared

likelihood = exp(-1/2*NIS)/(sqrt((2*pi)^2*det(S)));
end

== matlab function simulation/DHT - TVKFs/TVKF2/Time Varying KF ==
  data: Ad input; Bd input; C input; Qd input; Rd input; y input; u input; ybar output; NIS output; likelihood output; xbarPrev input; xbar output; PbarPrev input; Pbar output
function [ybar, NIS, likelihood, xbar, Pbar] = fcn(Ad, Bd, C, Qd, Rd, ...
    y, u, xbarPrev, PbarPrev)

n = size(xbarPrev, 1);
I = eye(n);

xhat = Ad*xbarPrev + Bd*u; % Predicted states
Phat = Ad*PbarPrev*Ad' + Qd; % Predicted covariances
yhat = C*xhat; % Predicted measurements
v = y - yhat; % Innovation
S = C*Phat*C' + Rd; % Innovation covariance
L = Phat*C'*inv(S); % Kalman gain
xbar = xhat + L*v; % Update states
Pbar = (I - L*C)*Phat*(I - L*C)' + L*Rd*L'; % Update covariances
ybar = C*xbar; % Updated measurements
NIS = v'*inv(S)*v; % Normalized innovations squared

likelihood = exp(-1/2*NIS)/(sqrt((2*pi)^2*det(S)));
end

== matlab function simulation/DHT - TVKFs/TVKF3/Time Varying KF ==
  data: Ad input; Bd input; C input; Qd input; Rd input; y input; u input; ybar output; NIS output; likelihood output; xbarPrev input; xbar output; PbarPrev input; Pbar output
function [ybar, NIS, likelihood, xbar, Pbar] = fcn(Ad, Bd, C, Qd, Rd, ...
    y, u, xbarPrev, PbarPrev)
n = size(xbarPrev, 1); 

I = eye(n);

xhat = Ad*xbarPrev + Bd*u; % Predicted states
Phat = Ad*PbarPrev*Ad' + Qd; % Predicted covariances
yhat = C*xhat; % Predicted measurements
v = y - yhat; % Innovation
S = C*Phat*C' + Rd; % Innovation covariance
L = Phat*C'*inv(S); % Kalman gain
xbar = xhat + L*v; % Update states
Pbar = (I - L*C)*Phat*(I - L*C)' + L*Rd*L'; % Update covariances
ybar = C*xbar; % Updated measurements
NIS = v'*inv(S)*v; % Normalized innovations squared

likelihood = exp(-1/2*NIS)/(sqrt((2*pi)^2*det(S)));
end
